simulink model "SimuRampaDiscreto"  (R2020a)
settings: Solver=VariableStepAuto  StartTime=0.0  StopTime=2  RelTol=1e-3
undefined symbols (not defined in the file): den, num, q0g1, q1g1, q2g1, q3g1, q4g1, s0g1, s1g1, Tm
libraries: simulink x1
settings Model: Creator=Alexander  LastModifiedBy=AsusPC
settings DataIOCC: ReturnWorkspaceOutputs=off
settings DebuggingCC: ArithmeticOperatorsInVariantConditions=warning
settings SFSimCC: SimUseLocalCustomCode=off  CustomCodeUndefinedFunction=UseInterfaceOnly
settings RTWCC: RTWUseLocalCustomCode=off

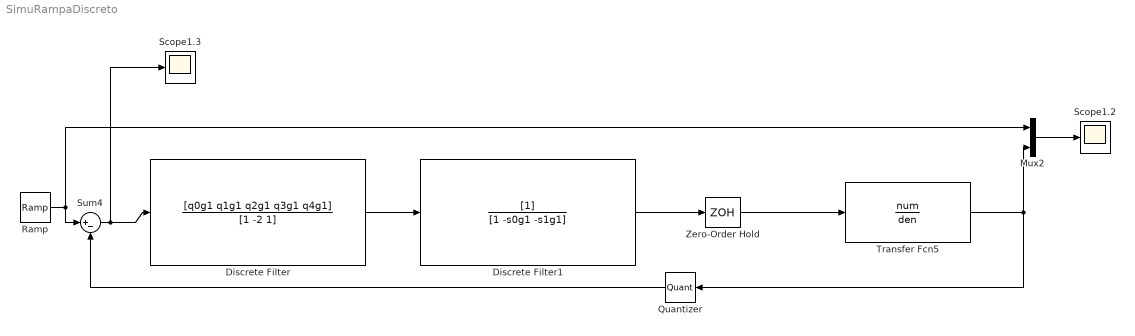
== system SimuRampaDiscreto ==
  Discrete Filter : DiscreteFilter  Numerator=[q0g1 q1g1 q2g1 q3g1 q4g1]  Denominator=[1 -2 1]  SampleTime=Tm
  Discrete Filter1 : DiscreteFilter  Denominator=[1 -s0g1 -s1g1]  SampleTime=Tm
  Mux2 : Mux  Inputs=2
  Quantizer : Quantizer  QuantizationInterval=3.3/1024
  Ramp : simulink/Sources/Ramp  slope=1  start=0  InitialOutput=0
  Scope1.2 : Scope
  Scope1.3 : Scope
  Sum4 : Sum  Inputs=|+-
  Transfer Fcn5 : TransferFcn  Numerator=num  Denominator=den
  Zero-Order Hold : ZeroOrderHold  SampleTime=Tm
  wires:
  Sum4/1 -> Scope1.3/1, Discrete Filter/1
  Transfer Fcn5/1 -> Mux2/2, Quantizer/1
  Mux2/1 -> Scope1.2/1
  Ramp/1 -> Mux2/1, Sum4/1
  Quantizer/1 -> Sum4/2
  Zero-Order Hold/1 -> Transfer Fcn5/1
  Discrete Filter/1 -> Discrete Filter1/1
  Discrete Filter1/1 -> Zero-Order Hold/1
